simulink model "pid_control_sim"  (R2019b)
settings: Solver=FixedStepAuto  StartTime=0.0  StopTime=69.8  FixedStep=h  RelTol=1e-3
values from neighbouring files (symbols this model uses):
  h = 0.1    [Example_9_Tracking_Delta_Input_Formulation.m]    (also in dyn_dist_mpc_control.m = 0.01; dyn_mpc_control.m = 0.01; dyn_pid_control.m = 0.01; init.m = 0.05)
  Kd = 5.6913    [dyn_pid_control.m]    (also in pid_control.m = 41.429)
  Ki = 1.9187    [dyn_pid_control.m]    (also in pid_control.m = 0.315)
  Kp = 23.086    [dyn_pid_control.m]    (also in pid_control.m = 34.37)
  robot_sys_ss = lateral_2_dof_model_continuous_time(h, robot_vel, 0)    [Example_9_Tracking_Delta_Input_Formulation.m]    (also in dyn_dist_mpc_control.m = c2d(robot_sys_ss, h); dyn_mpc_control.m = c2d(robot_sys_ss, h); mpc_control.m = c2d(robot_sys_ss, h); pid_control.m = c2d(robot_sys_ss, h))
  Tf = 0.053    [pid_control.m]
libraries: simulink x1
settings Model: Creator=faaizz  LastModifiedBy=faaizz
settings SFSimCC: CustomCodeUndefinedFunction=UseInterfaceOnly

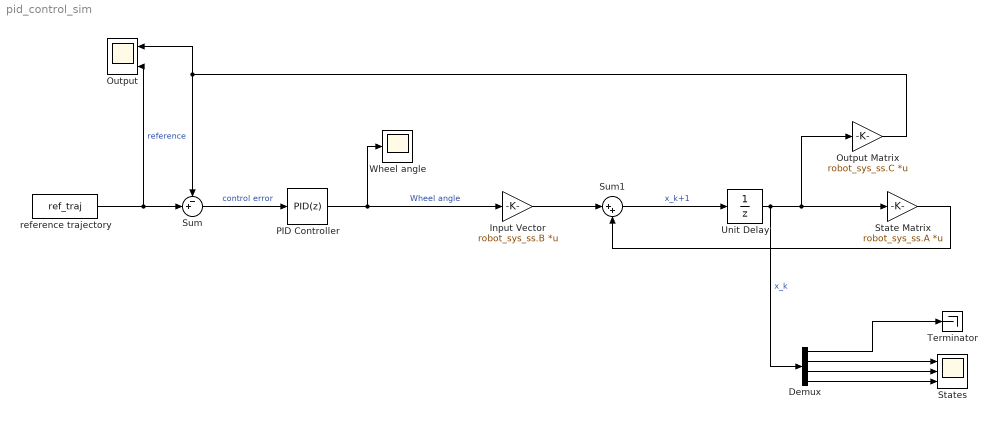
== system pid_control_sim ==
  Demux : Demux
  Input Vector : Gain  Gain=robot_sys_ss.B  Multiplication=Matrix(K*u)
  Output : Scope  NumInputPorts=2
  Output Matrix : Gain  Gain=robot_sys_ss.C  Multiplication=Matrix(K*u)
  PID Controller : simulink/Continuous/PID Controller  Controller=PID  Form=Parallel  TimeDomain=Discrete-time  SampleTime=h  IntegratorMethod=Forward Euler  FilterMethod=Forward Euler  ControllerParametersSource=internal  P=Kp  I=Ki  D=Kd  UseFilter=on  N=Tf  TunerSelectOption=Transfer Function Based (PID Tuner App)  InitialConditionSource=internal  InitialConditionForIntegrator=0  InitialConditionForFilter=0  DifferentiatorICPrevScaledInput=0  ExternalReset=none  TrackingMode=off  Kt=1  LimitOutput=off  UpperSaturationLimit=inf  LowerSaturationLimit=-inf  LinearizeAsGain=on  AntiWindupMode=none  Kb=1  POutMin=[]  POutMax=[]  IOutMin=[]  IOutMax=[]  DOutMin=[]  DOutMax=[]  NOutMin=[]  NOutMax=[]  SumOutMin=[]  SumOutMax=[]  SaturationOutMin=[]  SaturationOutMax=[]  PParamMin=[]  PParamMax=[]  IParamMin=[]  IParamMax=[]  DParamMin=[]  DParamMax=[]  NParamMin=[]  NParamMax=[]  KbParamMin=[]  KbParamMax=[]  KtParamMin=[]  KtParamMax=[]  KbOutMin=[]  KbOutMax=[]  KtOutMin=[]  KtOutMax=[]  IntegratorOutMin=[]  IntegratorOutMax=[]  FilterOutMin=[]  FilterOutMax=[]  SumI1OutMin=[]  SumI1OutMax=[]  SumI2OutMin=[]  SumI2OutMax=[]  SumI3OutMin=[]  SumI3OutMax=[]  SumI4OutMin=[]  SumI4OutMax=[]  SumDOutMin=[]  SumDOutMax=[]  DifferentiatorOutMin=[]  DifferentiatorOutMax=[]  FilterDiffOutCoefMin=[]  FilterDiffOutCoefMax=[]  ReciprocalOutMin=[]  ReciprocalOutMax=[]  SumDenOutMin=[]  SumDenOutMax=[]  SumNumOutMin=[]  SumNumOutMax=[]  DivideOutMin=[]  DivideOutMax=[]  IntegratorContinuousStateAttributes=''  IntegratorStateMustResolveToSignalObject=off  IntegratorRTWStateStorageClass=Auto  FilterContinuousStateAttributes=''  FilterStateMustResolveToSignalObject=off  FilterRTWStateStorageClass=Auto  ParallelPVariant=InternalParameters  IdealPVariant=Disabled  IVariant=InternalParameters  DVariant=InternalParameters  IntegratorVariant=Discrete  SatVariant=Disabled  AWVariant=Passthrough  PCopyVariant=Disabled  TRVariant=Disabled  FdbkBlocksVariant=Forward  IdealPFdbkVariant=Disabled  SatFdbkVariant=Disabled  DerivativeFilterVariant=ForwardEulerFilter  NVariant=InternalParameters  NCopyVariant=Disabled  FilterICVariant=InternalICsFilter  IntegratorICVariant=InternalICs  ExternalResetVariant=Disabled  TRSumVariant=Passthrough  SumFdbkVariant=Disabled  SumVariant=Sum_PID
  State Matrix : Gain  Gain=robot_sys_ss.A  Multiplication=Matrix(K*u)
  States : Scope  NumInputPorts=3
  Sum : Sum  Inputs=-+|
  Sum1 : Sum  Inputs=|++
  Terminator : Terminator
  Unit Delay : UnitDelay  SampleTime=-1  HasFrameUpgradeWarning=on
  Wheel angle : Scope
  reference trajectory : FromWorkspace  VariableName=ref_traj  SampleTime=0  OutputAfterFinalValue=Setting to zero
  wires:
  reference trajectory/1 -> Sum/2, Output/2  "reference"
  Sum/1 -> PID Controller/1  "control error"
  PID Controller/1 -> Input Vector/1, Wheel angle/1  "Wheel angle"
  Output Matrix/1 -> Output/1, Sum/1
  State Matrix/1 -> Sum1/2
  Sum1/1 -> Unit Delay/1  "x_k+1"
  Unit Delay/1 -> Demux/1, State Matrix/1, Output Matrix/1  "x_k"
  Demux/4 -> States/3
  Input Vector/1 -> Sum1/1
  Demux/1 -> Terminator/1
  Demux/3 -> States/2
  Demux/2 -> States/1
